simulink model "chap04_CA2"  (R2021a)
settings: Solver=FixedStepDiscrete  StartTime=0.0  StopTime=30  FixedStep=0.001  RelTol=1e-3
undefined symbols (not defined in the file): DiscIntNeverNeededParam
libraries: simulink x4
(part 1 of 3)
settings Model: Creator=陈天兴  LastModifiedBy=陈天兴

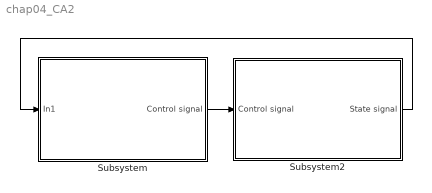
== system chap04_CA2 ==
  Subsystem : Subsystem
  Subsystem2 : Subsystem
  wires:
  Subsystem/1(Control signal) -> Subsystem2/1(Control signal)
  Subsystem2/1(State signal) -> Subsystem/1(In1)

== system chap04_CA2/Subsystem ==
  In1 : Inport
  Bus Creator : BusCreator  Inputs=6
  Bus Creator2 : BusCreator  Inputs=2
  Subsystem : Subsystem
  Subsystem1 : Subsystem
  Subsystem2 : Subsystem
  Subsystem3 : Subsystem
  Subsystem4 : Subsystem
  Subsystem5 : Subsystem
  Control signal : Outport
  wires:
  Bus Creator2/1 -> Subsystem/1(In19), Subsystem2/1(In19), Subsystem5/1(In19), Subsystem4/1(In19), Subsystem1/1(In19), Subsystem3/1(In19)
  Subsystem5/1(u3) -> Bus Creator/3
  Subsystem3/1(u4) -> Bus Creator/4
  Subsystem1/1(u5) -> Bus Creator/5
  Subsystem/1(u1) -> Bus Creator/1
  Subsystem2/1(u2) -> Bus Creator/2
  Subsystem4/1(u6) -> Bus Creator/6
  Bus Creator/1 -> [control], Control signal/1
  In1/1 -> Bus Creator2/1  "state(t)"
  [control] -> Bus Creator2/2  "control"

== system chap04_CA2/Subsystem2 ==
  Control signal : Inport
  Bus Creator : BusCreator  Inputs=7
  Bus Creator1 : BusCreator  Inputs=6
  Bus Selector : BusSelector  OutputSignals=node1.ux,node1.uy,node1.uz
  Bus Selector1 : BusSelector  OutputSignals=node2.ux,node2.uy,node2.uz
  Bus Selector2 : BusSelector  OutputSignals=node3.ux,node3.uy,node3.uz
  Bus Selector3 : BusSelector  OutputSignals=node4.ux,node4.uy,node4.uz
  Bus Selector4 : BusSelector  OutputSignals=node5.ux,node5.uy,node5.uz
  Bus Selector5 : BusSelector  OutputSignals=node6.ux,node6.uy,node6.uz
  Constant2 : Constant
  Scope : Scope  NumInputPorts=3
  Subsystem : Subsystem
  Subsystem1 : Subsystem
  Subsystem2 : Subsystem
  Subsystem3 : Subsystem
  Subsystem4 : Subsystem
  Subsystem5 : Subsystem
  Subsystem6 : Subsystem
  Subsystem7 : Subsystem
  State signal : Outport
  wires:
  Bus Creator/1 -> State signal/1
  Control signal/1 -> Bus Selector/1, Bus Selector1/1, Bus Selector5/1, Bus Selector4/1, Bus Selector3/1, Bus Selector2/1
  Bus Selector/1 -> Subsystem/4(ut1x)  "<ux>"
  Bus Selector/2 -> Subsystem/5(ut1y)  "<uy>"
  Bus Selector/3 -> Subsystem/6(ut1z)  "<uz>"
  Bus Selector1/1 -> Subsystem1/4(ut2x)  "<ux>"
  Bus Selector1/2 -> Subsystem1/5(ut2y)  "<uy>"
  Bus Selector1/3 -> Subsystem1/6(ut2z)  "<uz>"
  Bus Selector2/1 -> Subsystem2/4(ut3x)  "<ux>"
  Bus Selector2/2 -> Subsystem2/5(ut3y)  "<uy>"
  Bus Selector2/3 -> Subsystem2/6(ut3z)  "<uz>"
  Bus Selector3/1 -> Subsystem3/4(ut4x)  "<ux>"
  Bus Selector3/2 -> Subsystem3/5(ut4y)  "<uy>"
  Bus Selector3/3 -> Subsystem3/6(ut4z)  "<uz>"
  Bus Selector4/1 -> Subsystem4/4(ut5x)  "<ux>"
  Bus Selector4/2 -> Subsystem4/5(ut5y)  "<uy>"
  Bus Selector4/3 -> Subsystem4/6(ut5z)  "<uz>"
  Bus Selector5/1 -> Subsystem5/4(ut6x)  "<ux>"
  Bus Selector5/2 -> Subsystem5/5(ut6y)  "<uy>"
  Bus Selector5/3 -> Subsystem5/6(ut6z)  "<uz>"
  Subsystem5/1(node6) -> Bus Creator/7
  Subsystem4/1(node5) -> Bus Creator/6
  Subsystem3/1(node4) -> Bus Creator/5
  Subsystem2/1(node3) -> Bus Creator/4
  Subsystem1/1(node2) -> Bus Creator/3
  Subsystem/1(node1) -> Bus Creator/2
  Subsystem6/5(vy) -> Bus Creator1/5  "vy"
  Subsystem6/2(xy) -> Bus Creator1/2  "xy"
  Subsystem6/3(xz) -> Bus Creator1/3  "xz"
  Subsystem6/4(vx) -> Bus Creator1/4  "vx"
  Subsystem6/6(vz) -> Bus Creator1/6  "vz"
  Bus Creator1/1 -> Bus Creator/1  "node0"
  Subsystem6/1(xx) -> Bus Creator1/1  "xx"
  Subsystem7/2(dy) -> Subsystem/2(dy), Subsystem5/2(dy), Subsystem4/2(dy), Subsystem3/2(dy), Subsystem2/2(dy), Subsystem1/2(dy), Scope/2  "dy"
  Subsystem7/3(dz) -> Subsystem5/3(dz), Subsystem4/3(dz), Subsystem3/3(dz), Subsystem2/3(dz), Subsystem1/3(dz), Subsystem/3(dz), Scope/3  "dz"
  Subsystem7/1(dx) -> Subsystem3/1(dx), Subsystem5/1(dx), Subsystem4/1(dx), Subsystem2/1(dx), Subsystem1/1(dx), Subsystem/1(dx), Scope/1  "dx"
  Constant2/1 -> Subsystem7/1(switch)

== system chap04_CA2/Subsystem/Subsystem ==
  In19 : Inport
  Bus Creator : BusCreator  Inputs=3
  Bus Selector : BusSelector  OutputSignals=state(t).node1.xx,state(t).node2.xx,state(t).node3.xx,state(t).node6.xx,state(t).node1.vx,state(t).node2.vx,state(t).node3.vx,state(t).node6.vx
  Bus Selector1 : BusSelector  OutputSignals=state(t).node1.xy,state(t).node2.xy,state(t).node3.xy,state(t).node6.xy,state(t).node1.vy,state(t).node2.vy,state(t).node3.vy,state(t).node6.vy
  Bus Selector2 : BusSelector  OutputSignals=state(t).node1.xz,state(t).node2.xz,state(t).node3.xz,state(t).node6.xz,state(t).node1.vz,state(t).node2.vz,state(t).node3.vz,state(t).node6.vz
  Bus Selector3 : BusSelector  OutputSignals=state(t).node1.vx
  Bus Selector4 : BusSelector  OutputSignals=state(t).node1.vy
  Bus Selector5 : BusSelector  OutputSignals=state(t).node1.vz
  Constant : Constant  Value=1.5
  Subsystem1 : Subsystem
  Subsystem10 : Subsystem
  Subsystem2 : Subsystem
  Subsystem4 : Subsystem
  Subsystem6 : Subsystem
  Subsystem7 : Subsystem
  Subsystem8 : Subsystem
  u1 : Outport
  wires:
  Subsystem2/1(utx) -> Subsystem8/2(utz)
  Subsystem6/1(utx) -> Subsystem4/2(utx)
  Subsystem1/1(utx) -> Subsystem7/2(uty)
  Bus Creator/1 -> u1/1  "node1"
  [state] -> Bus Selector3/1
  Bus Selector3/1 -> Subsystem4/1(vx1)  "<vx>"
  Bus Selector4/1 -> Subsystem7/1(vy1)  "<vy>"
  [state] -> Bus Selector4/1
  [state] -> Bus Selector5/1
  Bus Selector5/1 -> Subsystem8/1(vz1)  "<vz>"
  [gain] -> Subsystem8/3(gain)
  [gain] -> Subsystem7/3(gain)
  [gain] -> Subsystem4/3(gain)
  Subsystem10/1(ux) -> Bus Creator/1  "ux"
  Subsystem10/2(uy) -> Bus Creator/2  "uy"
  Subsystem10/3(uz) -> Bus Creator/3  "uz"
  In19/1 -> Bus Selector1/1, Bus Selector/1, Bus Selector2/1, [state]
  Bus Selector1/2 -> Subsystem1/2(xy2)  "<xy>"
  Bus Selector/2 -> Subsystem6/2(xx2)  "<xx>"
  Bus Selector/7 -> Subsystem6/7(vx3)  "<vx>"
  Bus Selector2/3 -> Subsystem2/3(xz3)  "<xz>"
  Bus Selector2/6 -> Subsystem2/6(vz2)  "<vz>"
  Bus Selector2/7 -> Subsystem2/7(vz3)  "<vz>"
  Bus Selector/1 -> Subsystem6/1(xx1)  "<xx>"
  Bus Selector1/4 -> Subsystem1/4(xy6)  "<xy>"
  Bus Selector2/5 -> Subsystem2/5(vz1)  "<vz>"
  Bus Selector2/4 -> Subsystem2/4(xz6)  "<xz>"
  Bus Selector/6 -> Subsystem6/6(vx2)  "<vx>"
  Bus Selector1/1 -> Subsystem1/1(xy1)  "<xy>"
  Bus Selector2/8 -> Subsystem2/8(vz6)  "<vz>"
  Bus Selector2/1 -> Subsystem2/1(xz1)  "<xz>"
  Bus Selector2/2 -> Subsystem2/2(xx2)  "<xz>"
  Bus Selector1/8 -> Subsystem1/8(vy6)  "<vy>"
  Bus Selector1/7 -> Subsystem1/7(vy3)  "<vy>"
  Bus Selector1/3 -> Subsystem1/3(xy3)  "<xy>"
  Bus Selector1/5 -> Subsystem1/5(vy1)  "<vy>"
  Bus Selector1/6 -> Subsystem1/6(vy2)  "<vy>"
  Bus Selector/5 -> Subsystem6/5(vx1)  "<vx>"
  Bus Selector/4 -> Subsystem6/4(xx6)  "<xx>"
  Bus Selector/3 -> Subsystem6/3(xx3)  "<xx>"
  Bus Selector/8 -> Subsystem6/8(vx6)  "<vx>"
  Subsystem7/1(ux) -> Subsystem10/2(uty)
  Subsystem4/1(ux) -> Subsystem10/1(utx)
  Subsystem8/1(ux) -> Subsystem10/3(utz)
  Constant/1 -> [gain]

== system chap04_CA2/Subsystem/Subsystem1 ==
  In19 : Inport
  Bus Creator : BusCreator  Inputs=3
  Bus Selector : BusSelector  OutputSignals=state(t).node5.xx,state(t).node0.xx,state(t).node3.xx,state(t).node4.xx,state(t).node5.vx,state(t).node0.vx,state(t).node3.vx,state(t).node4.vx
  Bus Selector1 : BusSelector  OutputSignals=state(t).node5.xy,state(t).node0.xy,state(t).node3.xy,state(t).node4.xy,state(t).node5.vy,state(t).node0.vy,state(t).node3.vy,state(t).node4.vy
  Bus Selector2 : BusSelector  OutputSignals=state(t).node5.xz,state(t).node0.xz,state(t).node3.xz,state(t).node4.xz,state(t).node5.vz,state(t).node0.vz,state(t).node3.vz,state(t).node4.vz
  Bus Selector3 : BusSelector  OutputSignals=state(t).node5.vx,state(t).node0.vx
  Bus Selector4 : BusSelector  OutputSignals=state(t).node5.vy,state(t).node0.vx
  Bus Selector5 : BusSelector  OutputSignals=state(t).node5.vz,state(t).node0.vz
  Constant : Constant  Value=1.5
  Subsystem1 : Subsystem
  Subsystem10 : Subsystem
  Subsystem2 : Subsystem
  Subsystem4 : Subsystem
  Subsystem6 : Subsystem
  Subsystem7 : Subsystem
  Subsystem8 : Subsystem
  u5 : Outport
  wires:
  Bus Creator/1 -> u5/1  "node5"
  Subsystem10/3(uz) -> Bus Creator/3  "uz"
  Subsystem10/2(uy) -> Bus Creator/2  "uy"
  Subsystem10/1(ux) -> Bus Creator/1  "ux"
  [gain] -> Subsystem8/4(gain)
  Subsystem2/1(utz) -> Subsystem8/3(utz)
  Subsystem1/1(uty) -> Subsystem7/3(uty)
  [state] -> Bus Selector3/1
  Bus Selector3/2 -> Subsystem4/2(vx0)  "<vx>"
  Bus Selector3/1 -> Subsystem4/1(vx5)  "<vx>"
  Bus Selector5/1 -> Subsystem8/1(vz5)  "<vz>"
  [state] -> Bus Selector4/1
  Subsystem6/1(utx) -> Subsystem4/3(utx)
  [state] -> Bus Selector5/1
  Bus Selector4/1 -> Subsystem7/1(vy5)  "<vy>"
  Bus Selector4/2 -> Subsystem7/2(vy0)  "<vx>"
  Bus Selector5/2 -> Subsystem8/2(vz0)  "<vz>"
  [gain] -> Subsystem4/4(gain)
  [gain] -> Subsystem7/4(gain)
  In19/1 -> Bus Selector/1, Bus Selector2/1, [state], Bus Selector1/1
  Bus Selector1/8 -> Subsystem1/8(vy4)  "<vy>"
  Bus Selector1/7 -> Subsystem1/7(vy3)  "<vy>"
  Bus Selector1/6 -> Subsystem1/6(vy0)  "<vy>"
  Bus Selector1/5 -> Subsystem1/5(vy5)  "<vy>"
  Bus Selector1/4 -> Subsystem1/4(xy4)  "<xy>"
  Bus Selector1/3 -> Subsystem1/3(xy3)  "<xy>"
  Bus Selector1/2 -> Subsystem1/2(xy0)  "<xy>"
  Bus Selector1/1 -> Subsystem1/1(xy5)  "<xy>"
  Bus Selector/8 -> Subsystem6/8(vx4)  "<vx>"
  Bus Selector/7 -> Subsystem6/7(vx3)  "<vx>"
  Bus Selector/6 -> Subsystem6/6(vx0)  "<vx>"
  Bus Selector/5 -> Subsystem6/5(vx5)  "<vx>"
  Bus Selector/4 -> Subsystem6/4(xx4)  "<xx>"
  Bus Selector/3 -> Subsystem6/3(xx3)  "<xx>"
  Bus Selector/2 -> Subsystem6/2(xx0)  "<xx>"
  Bus Selector/1 -> Subsystem6/1(xx5)  "<xx>"
  Bus Selector2/1 -> Subsystem2/1(xz5)  "<xz>"
  Bus Selector2/2 -> Subsystem2/2(xz0)  "<xz>"
  Bus Selector2/3 -> Subsystem2/3(xz3)  "<xz>"
  Bus Selector2/4 -> Subsystem2/4(xz4)  "<xz>"
  Bus Selector2/5 -> Subsystem2/5(vz5)  "<vz>"
  Bus Selector2/6 -> Subsystem2/6(vz0)  "<vz>"
  Bus Selector2/7 -> Subsystem2/7(vz3)  "<vz>"
  Bus Selector2/8 -> Subsystem2/8(vz4)  "<vz>"
  Subsystem7/1(ux) -> Subsystem10/2(uty)
  Subsystem8/1(ux) -> Subsystem10/3(utz)
  Subsystem4/1(ux) -> Subsystem10/1(utx)
  Constant/1 -> [gain]

== system chap04_CA2/Subsystem/Subsystem2 ==
  In19 : Inport
  Bus Creator : BusCreator  Inputs=3
  Bus Selector10 : BusSelector  OutputSignals=state(t).node2.xy,state(t).node1.xy,state(t).node4.xy,state(t).node6.xy,state(t).node2.vy,state(t).node1.vy,state(t).node4.vy,state(t).node6.vy
  Bus Selector11 : BusSelector  OutputSignals=state(t).node2.xz,state(t).node1.xz,state(t).node4.xz,state(t).node6.xz,state(t).node2.vz,state(t).node1.vz,state(t).node4.vz,state(t).node6.vz
  Bus Selector3 : BusSelector  OutputSignals=state(t).node2.vx
  Bus Selector4 : BusSelector  OutputSignals=state(t).node2.vy
  Bus Selector5 : BusSelector  OutputSignals=state(t).node2.vz
  Bus Selector9 : BusSelector  OutputSignals=state(t).node2.xx,state(t).node1.xx,state(t).node4.xx,state(t).node6.xx,state(t).node2.vx,state(t).node1.vx,state(t).node4.vx,state(t).node6.vx
  Constant : Constant  Value=1.5
  Subsystem1 : Subsystem
  Subsystem10 : Subsystem
  Subsystem2 : Subsystem
  Subsystem4 : Subsystem
  Subsystem6 : Subsystem
  Subsystem7 : Subsystem
  Subsystem8 : Subsystem
  u2 : Outport
  wires:
  Bus Creator/1 -> u2/1  "node2"
  Subsystem10/1(ux) -> Bus Creator/1  "ux"
  Subsystem10/2(uy) -> Bus Creator/2  "uy"
  Subsystem10/3(uz) -> Bus Creator/3  "uz"
  Subsystem1/1(p2y) -> Subsystem7/2(uty)
  [state] -> Bus Selector4/1
  Subsystem2/1(p2z) -> Subsystem8/2(utz)
  Bus Selector4/1 -> Subsystem7/1(vy1)  "<vy>"
  Bus Selector5/1 -> Subsystem8/1(vz1)  "<vz>"
  [gain] -> Subsystem8/3(gain)
  [gain] -> Subsystem4/3(gain)
  [gain] -> Subsystem7/3(gain)
  [state] -> Bus Selector3/1
  Subsystem6/1(p2x) -> Subsystem4/2(utx)
  Bus Selector3/1 -> Subsystem4/1(vx1)  "<vx>"
  [state] -> Bus Selector5/1
  Bus Selector11/8 -> Subsystem2/8(vz6)  "<vz>"
  Bus Selector11/7 -> Subsystem2/7(vz4)  "<vz>"
  Bus Selector11/6 -> Subsystem2/6(vz1)  "<vz>"
  Bus Selector11/5 -> Subsystem2/5(vz2)  "<vz>"
  Bus Selector11/4 -> Subsystem2/4(xz6)  "<xz>"
  Bus Selector11/3 -> Subsystem2/3(xz4)  "<xz>"
  Bus Selector11/2 -> Subsystem2/2(xz1)  "<xz>"
  Bus Selector11/1 -> Subsystem2/1(xz2)  "<xz>"
  Bus Selector10/8 -> Subsystem1/8(vy6)  "<vy>"
  Bus Selector10/7 -> Subsystem1/7(vy4)  "<vy>"
  Bus Selector10/6 -> Subsystem1/6(vy1)  "<vy>"
  Bus Selector10/5 -> Subsystem1/5(vy2)  "<vy>"
  Bus Selector10/4 -> Subsystem1/4(xy6)  "<xy>"
  Bus Selector10/3 -> Subsystem1/3(xy4)  "<xy>"
  Bus Selector10/2 -> Subsystem1/2(xy1)  "<xy>"
  Bus Selector10/1 -> Subsystem1/1(xy2)  "<xy>"
  Bus Selector9/1 -> Subsystem6/1(xx2)  "<xx>"
  Bus Selector9/2 -> Subsystem6/2(xx1)  "<xx>"
  Bus Selector9/3 -> Subsystem6/3(xx4)  "<xx>"
  Bus Selector9/4 -> Subsystem6/4(xx6)  "<xx>"
  Bus Selector9/5 -> Subsystem6/5(vx2)  "<vx>"
  Bus Selector9/6 -> Subsystem6/6(vx1)  "<vx>"
  Bus Selector9/7 -> Subsystem6/7(vx4)  "<vx>"
  Bus Selector9/8 -> Subsystem6/8(vx6)  "<vx>"
  In19/1 -> [state], Bus Selector11/1, Bus Selector9/1, Bus Selector10/1
  Subsystem7/1(ux) -> Subsystem10/2(uty)
  Subsystem8/1(ux) -> Subsystem10/3(utz)
  Subsystem4/1(ux) -> Subsystem10/1(utx)
  Constant/1 -> [gain]

== system chap04_CA2/Subsystem/Subsystem3 ==
  In19 : Inport
  Bus Creator : BusCreator  Inputs=3
  Bus Selector : BusSelector  OutputSignals=state(t).node4.xx,state(t).node2.xx,state(t).node3.xx,state(t).node5.xx,state(t).node4.vx,state(t).node2.vx,state(t).node3.vx,state(t).node5.vx
  Bus Selector1 : BusSelector  OutputSignals=state(t).node4.xy,state(t).node2.xy,state(t).node3.xy,state(t).node5.xy,state(t).node4.vy,state(t).node2.vy,state(t).node3.vy,state(t).node5.vy
  Bus Selector2 : BusSelector  OutputSignals=state(t).node4.xz,state(t).node2.xz,state(t).node3.xz,state(t).node5.xz,state(t).node4.vz,state(t).node2.vz,state(t).node3.vz,state(t).node5.vz
  Bus Selector3 : BusSelector  OutputSignals=state(t).node4.vx
  Bus Selector4 : BusSelector  OutputSignals=state(t).node4.vy
  Bus Selector5 : BusSelector  OutputSignals=state(t).node4.vz
  Constant : Constant  Value=1.5
  Subsystem1 : Subsystem
  Subsystem10 : Subsystem
  Subsystem2 : Subsystem
  Subsystem4 : Subsystem
  Subsystem6 : Subsystem
  Subsystem7 : Subsystem
  Subsystem8 : Subsystem
  u4 : Outport
  wires:
  Bus Creator/1 -> u4/1  "node4"
  [state] -> Bus Selector5/1
  Subsystem2/1(utx) -> Subsystem8/2(utz)
  Bus Selector5/1 -> Subsystem8/1(vz4)  "<vz>"
  [state] -> Bus Selector4/1
  [gain] -> Subsystem8/3(gain)
  Subsystem6/1(utx) -> Subsystem4/2(utx)
  Bus Selector4/1 -> Subsystem7/1(vy4)  "<vy>"
  Subsystem1/1(utx) -> Subsystem7/2(uty)
  Bus Selector3/1 -> Subsystem4/1(vx4)  "<vx>"
  [gain] -> Subsystem7/3(gain)
  [gain] -> Subsystem4/3(gain)
  [state] -> Bus Selector3/1
  Subsystem10/1(ux) -> Bus Creator/1  "ux"
  Subsystem10/2(uy) -> Bus Creator/2  "uy"
  Subsystem10/3(uz) -> Bus Creator/3  "uz"
  Bus Selector1/6 -> Subsystem1/6(vy2)  "<vy>"
  Bus Selector/6 -> Subsystem6/6(vx2)  "<vx>"
  In19/1 -> Bus Selector/1, Bus Selector1/1, Bus Selector2/1, [state]
  Bus Selector/7 -> Subsystem6/7(vx3)  "<vx>"
  Bus Selector1/2 -> Subsystem1/2(xy2)  "<xy>"
  Bus Selector2/3 -> Subsystem2/3(xz3)  "<xz>"
  Bus Selector1/3 -> Subsystem1/3(xy3)  "<xy>"
  Bus Selector2/1 -> Subsystem2/1(xz4)  "<xz>"
  Bus Selector1/1 -> Subsystem1/1(xy4)  "<xy>"
  Bus Selector/3 -> Subsystem6/3(xx3)  "<xx>"
  Bus Selector/1 -> Subsystem6/1(xx4)  "<xx>"
  Bus Selector/8 -> Subsystem6/8(vx5)  "<vx>"
  Bus Selector1/4 -> Subsystem1/4(xy5)  "<xy>"
  Bus Selector/4 -> Subsystem6/4(xx5)  "<xx>"
  Bus Selector/5 -> Subsystem6/5(vx4)  "<vx>"
  Bus Selector1/7 -> Subsystem1/7(vy3)  "<vy>"
  Bus Selector2/7 -> Subsystem2/7(vz3)  "<vz>"
  Bus Selector2/4 -> Subsystem2/4(xz5)  "<xz>"
  Bus Selector2/8 -> Subsystem2/8(vz5)  "<vz>"
  Bus Selector1/8 -> Subsystem1/8(vy5)  "<vy>"
  Bus Selector/2 -> Subsystem6/2(xx2)  "<xx>"
  Bus Selector2/2 -> Subsystem2/2(xx2)  "<xz>"
  Bus Selector1/5 -> Subsystem1/5(vy4)  "<vy>"
  Bus Selector2/5 -> Subsystem2/5(vz4)  "<vz>"
  Bus Selector2/6 -> Subsystem2/6(vz2)  "<vz>"
  Subsystem4/1(ux) -> Subsystem10/1(utx)
  Subsystem8/1(ux) -> Subsystem10/3(utz)
  Subsystem7/1(ux) -> Subsystem10/2(uty)
  Constant/1 -> [gain]

== system chap04_CA2/Subsystem/Subsystem4 ==
  In19 : Inport
  Bus Creator : BusCreator  Inputs=3
  Bus Selector : BusSelector  OutputSignals=state(t).node6.xx,state(t).node0.xx,state(t).node1.xx,state(t).node2.xx,state(t).node6.vx,state(t).node0.vx,state(t).node1.vx,state(t).node2.vx
  Bus Selector1 : BusSelector  OutputSignals=state(t).node6.xy,state(t).node0.xy,state(t).node1.xy,state(t).node2.xy,state(t).node6.vy,state(t).node0.vy,state(t).node1.vy,state(t).node2.vy
  Bus Selector2 : BusSelector  OutputSignals=state(t).node6.xz,state(t).node0.xz,state(t).node1.xz,state(t).node2.xz,state(t).node6.vz,state(t).node0.vz,state(t).node1.vz,state(t).node2.vz
  Bus Selector3 : BusSelector  OutputSignals=state(t).node6.vx,state(t).node0.vx
  Bus Selector4 : BusSelector  OutputSignals=state(t).node6.vy,state(t).node0.vx
  Bus Selector5 : BusSelector  OutputSignals=state(t).node6.vz,state(t).node0.vz
  Constant : Constant  Value=1.5
  Subsystem1 : Subsystem
  Subsystem10 : Subsystem
  Subsystem2 : Subsystem
  Subsystem4 : Subsystem
  Subsystem6 : Subsystem
  Subsystem7 : Subsystem
  Subsystem8 : Subsystem
  u6 : Outport
  wires:
  Bus Creator/1 -> u6/1  "node6"
  Subsystem10/3(uz) -> Bus Creator/3  "uz"
  Subsystem10/2(uy) -> Bus Creator/2  "uy"
  Subsystem10/1(ux) -> Bus Creator/1  "ux"
  Bus Selector5/2 -> Subsystem8/2(vz0)  "<vz>"
  [gain] -> Subsystem7/4(gain)
  Subsystem1/1(utx) -> Subsystem7/3(uty)
  Subsystem2/1(utx) -> Subsystem8/3(utz)
  [state] -> Bus Selector3/1
  Bus Selector5/1 -> Subsystem8/1(vz6)  "<vz>"
  Bus Selector4/2 -> Subsystem7/2(vy0)  "<vx>"
  [gain] -> Subsystem4/4(gain)
  [state] -> Bus Selector5/1
  Subsystem6/1(utx) -> Subsystem4/3(utx)
  Bus Selector3/1 -> Subsystem4/1(vx6)  "<vx>"
  Bus Selector3/2 -> Subsystem4/2(vx0)  "<vx>"
  [gain] -> Subsystem8/4(gain)
  [state] -> Bus Selector4/1
  Bus Selector4/1 -> Subsystem7/1(vy6)  "<vy>"
  In19/1 -> Bus Selector/1, [state], Bus Selector2/1, Bus Selector1/1
  Bus Selector1/1 -> Subsystem1/1(xx6)  "<xy>"
  Bus Selector1/2 -> Subsystem1/2(xx0)  "<xy>"
  Bus Selector1/3 -> Subsystem1/3(xx1)  "<xy>"
  Bus Selector1/4 -> Subsystem1/4(xx2)  "<xy>"
  Bus Selector1/5 -> Subsystem1/5(vx6)  "<vy>"
  Bus Selector1/6 -> Subsystem1/6(vx0)  "<vy>"
  Bus Selector1/7 -> Subsystem1/7(vx1)  "<vy>"
  Bus Selector1/8 -> Subsystem1/8(vx2)  "<vy>"
  Bus Selector2/1 -> Subsystem2/1(xx6)  "<xz>"
  Bus Selector2/3 -> Subsystem2/3(xx1)  "<xz>"
  Bus Selector2/2 -> Subsystem2/2(xx0)  "<xz>"
  Bus Selector2/4 -> Subsystem2/4(xx2)  "<xz>"
  Bus Selector2/5 -> Subsystem2/5(vx6)  "<vz>"
  Bus Selector2/6 -> Subsystem2/6(vx0)  "<vz>"
  Bus Selector2/7 -> Subsystem2/7(vx1)  "<vz>"
  Bus Selector2/8 -> Subsystem2/8(vx2)  "<vz>"
  Bus Selector/8 -> Subsystem6/8(vx2)  "<vx>"
  Bus Selector/7 -> Subsystem6/7(vx1)  "<vx>"
  Bus Selector/6 -> Subsystem6/6(vx0)  "<vx>"
  Bus Selector/5 -> Subsystem6/5(vx6)  "<vx>"
  Bus Selector/4 -> Subsystem6/4(xx2)  "<xx>"
  Bus Selector/3 -> Subsystem6/3(xx1)  "<xx>"
  Bus Selector/2 -> Subsystem6/2(xx0)  "<xx>"
  Bus Selector/1 -> Subsystem6/1(xx6)  "<xx>"
  Subsystem7/1(ux) -> Subsystem10/2(uty)
  Subsystem8/1(ux) -> Subsystem10/3(utz)
  Subsystem4/1(ux) -> Subsystem10/1(utx)
  Constant/1 -> [gain]

== system chap04_CA2/Subsystem/Subsystem5 ==
  In19 : Inport
  Bus Creator : BusCreator  Inputs=3
  Bus Selector10 : BusSelector  OutputSignals=state(t).node3.xy,state(t).node1.xy,state(t).node4.xy,state(t).node5.xy,state(t).node3.vy,state(t).node1.vy,state(t).node4.vy,state(t).node5.vy
  Bus Selector11 : BusSelector  OutputSignals=state(t).node3.xz,state(t).node1.xz,state(t).node4.xz,state(t).node5.xz,state(t).node3.vz,state(t).node1.vz,state(t).node4.vz,state(t).node5.vz
  Bus Selector3 : BusSelector  OutputSignals=state(t).node3.vx
  Bus Selector4 : BusSelector  OutputSignals=state(t).node3.vy
  Bus Selector5 : BusSelector  OutputSignals=state(t).node3.vz
  Bus Selector9 : BusSelector  OutputSignals=state(t).node3.xx,state(t).node1.xx,state(t).node4.xx,state(t).node5.xx,state(t).node3.vx,state(t).node1.vx,state(t).node4.vx,state(t).node5.vx
  Constant : Constant  Value=1.5
  Subsystem1 : Subsystem
  Subsystem10 : Subsystem
  Subsystem2 : Subsystem
  Subsystem4 : Subsystem
  Subsystem6 : Subsystem
  Subsystem7 : Subsystem
  Subsystem8 : Subsystem
  u3 : Outport
  wires:
  Bus Creator/1 -> u3/1  "node3"
  Subsystem10/1(ux) -> Bus Creator/1  "ux"
  Subsystem10/2(uy) -> Bus Creator/2  "uy"
  Subsystem10/3(uz) -> Bus Creator/3  "uz"
  In19/1 -> Bus Selector9/1, Bus Selector10/1, [state], Bus Selector11/1
  Subsystem6/1(p3x) -> Subsystem4/2(utx)
  [gain] -> Subsystem7/3(gain)
  Bus Selector4/1 -> Subsystem7/1(vy3)  "<vy>"
  [state] -> Bus Selector5/1
  [state] -> Bus Selector3/1
  Bus Selector3/1 -> Subsystem4/1(vx3)  "<vx>"
  Bus Selector5/1 -> Subsystem8/1(vz3)  "<vz>"
  [gain] -> Subsystem4/3(gain)
  [gain] -> Subsystem8/3(gain)
  Subsystem2/1(p3z) -> Subsystem8/2(utz)
  Subsystem1/1(p3y) -> Subsystem7/2(uty)
  [state] -> Bus Selector4/1
  Bus Selector10/1 -> Subsystem1/1(xy3)  "<xy>"
  Bus Selector10/2 -> Subsystem1/2(xy1)  "<xy>"
  Bus Selector10/3 -> Subsystem1/3(xy4)  "<xy>"
  Bus Selector10/4 -> Subsystem1/4(xy5)  "<xy>"
  Bus Selector10/5 -> Subsystem1/5(vy3)  "<vy>"
  Bus Selector10/6 -> Subsystem1/6(vy1)  "<vy>"
  Bus Selector10/7 -> Subsystem1/7(vy4)  "<vy>"
  Bus Selector10/8 -> Subsystem1/8(vy5)  "<vy>"
  Bus Selector11/1 -> Subsystem2/1(xz3)  "<xz>"
  Bus Selector11/2 -> Subsystem2/2(xz1)  "<xz>"
  Bus Selector11/3 -> Subsystem2/3(xz4)  "<xz>"
  Bus Selector11/4 -> Subsystem2/4(xz5)  "<xz>"
  Bus Selector11/5 -> Subsystem2/5(vz3)  "<vz>"
  Bus Selector11/6 -> Subsystem2/6(vz1)  "<vz>"
  Bus Selector11/7 -> Subsystem2/7(vz4)  "<vz>"
  Bus Selector11/8 -> Subsystem2/8(vz5)  "<vz>"
  Bus Selector9/1 -> Subsystem6/1(xx3)  "<xx>"
  Bus Selector9/2 -> Subsystem6/2(xx1)  "<xx>"
  Bus Selector9/3 -> Subsystem6/3(xx4)  "<xx>"
  Bus Selector9/4 -> Subsystem6/4(xx5)  "<xx>"
  Bus Selector9/5 -> Subsystem6/5(vx3)  "<vx>"
  Bus Selector9/6 -> Subsystem6/6(vx1)  "<vx>"
  Bus Selector9/7 -> Subsystem6/7(vx4)  "<vx>"
  Bus Selector9/8 -> Subsystem6/8(vx5)  "<vx>"
  Subsystem7/1(ux) -> Subsystem10/2(uty)
  Subsystem8/1(ux) -> Subsystem10/3(utz)
  Subsystem4/1(ux) -> Subsystem10/1(utx)
  Constant/1 -> [gain]

== system chap04_CA2/Subsystem2/Subsystem ==
  dx : Inport
  dy : Inport  Port=2
  dz : Inport  Port=3
  ut1x : Inport  Port=4
  ut1y : Inport  Port=5
  ut1z : Inport  Port=6
  Add : Sum
  Add1 : Sum
  Add2 : Sum
  Add3 : Sum  Inputs=-+
  Add4 : Sum  Inputs=-+
  Add5 : Sum  Inputs=-+
  Bus Creator1 : BusCreator  Inputs=6
  Constant : Constant  Value=-1
  Constant1 : Constant
  Constant2 : Constant  Value=0
  Discrete-Time Integrator{,15..17} (4 alike) : DiscreteIntegrator  SampleTime=-1  ICPrevOutput=DiscIntNeverNeededParam  ICPrevScaledInput=DiscIntNeverNeededParam
  Discrete-Time Integrator14 : DiscreteIntegrator  InitialCondition=-1  SampleTime=-1  ICPrevOutput=DiscIntNeverNeededParam  ICPrevScaledInput=DiscIntNeverNeededParam
  Discrete-Time Integrator5 : DiscreteIntegrator  InitialCondition=1  SampleTime=-1  ICPrevOutput=DiscIntNeverNeededParam  ICPrevScaledInput=DiscIntNeverNeededParam
  node1 : Outport
  wires:
  ut1y/1 -> Add1/2
  ut1z/1 -> Add2/2
  Discrete-Time Integrator17/1 -> Discrete-Time Integrator15/1, Bus Creator1/5  "vy"
  Discrete-Time Integrator/1 -> Discrete-Time Integrator5/1, Bus Creator1/6  "vz"
  ut1x/1 -> Add/2
  Discrete-Time Integrator16/1 -> Bus Creator1/4, Discrete-Time Integrator14/1  "vx"
  Bus Creator1/1 -> node1/1  "node1"
  Add5/1 -> Bus Creator1/3  "xz"
  Add4/1 -> Bus Creator1/2  "xy"
  Add3/1 -> Bus Creator1/1  "xx"
  Add/1 -> Discrete-Time Integrator16/1
  Add1/1 -> Discrete-Time Integrator17/1
  Add2/1 -> Discrete-Time Integrator/1
  dy/1 -> Add1/1
  dz/1 -> Add2/1
  dx/1 -> Add/1
  Discrete-Time Integrator14/1 -> Add3/2
  Discrete-Time Integrator5/1 -> Add5/2
  Discrete-Time Integrator15/1 -> Add4/2
  Constant/1 -> Add3/1
  Constant1/1 -> Add4/1
  Constant2/1 -> Add5/1

== system chap04_CA2/Subsystem2/Subsystem1 ==
  dx : Inport
  dy : Inport  Port=2
  dz : Inport  Port=3
  ut2x : Inport  Port=4
  ut2y : Inport  Port=5
  ut2z : Inport  Port=6
  Add : Sum
  Add1 : Sum
  Add2 : Sum
  Add3 : Sum  Inputs=-+
  Add4 : Sum  Inputs=-+
  Add5 : Sum  Inputs=-+
  Bus Creator1 : BusCreator  Inputs=6
  Constant : Constant
  Constant1 : Constant
  Constant2 : Constant  Value=0
  Discrete-Time Integrator : DiscreteIntegrator  SampleTime=-1  ICPrevOutput=DiscIntNeverNeededParam  ICPrevScaledInput=DiscIntNeverNeededParam
  Discrete-Time Integrator14 : DiscreteIntegrator  InitialCondition=1.5  SampleTime=-1  ICPrevOutput=DiscIntNeverNeededParam  ICPrevScaledInput=DiscIntNeverNeededParam
  Discrete-Time Integrator15 : DiscreteIntegrator  InitialCondition=0.5  SampleTime=-1  ICPrevOutput=DiscIntNeverNeededParam  ICPrevScaledInput=DiscIntNeverNeededParam
  Discrete-Time Integrator16 : DiscreteIntegrator  SampleTime=-1  ICPrevOutput=DiscIntNeverNeededParam  ICPrevScaledInput=DiscIntNeverNeededParam
  Discrete-Time Integrator17 : DiscreteIntegrator  SampleTime=-1  ICPrevOutput=DiscIntNeverNeededParam  ICPrevScaledInput=DiscIntNeverNeededParam
  Discrete-Time Integrator5 : DiscreteIntegrator  InitialCondition=1  SampleTime=-1  ICPrevOutput=DiscIntNeverNeededParam  ICPrevScaledInput=DiscIntNeverNeededParam
  node2 : Outport
  wires:
  Bus Creator1/1 -> node2/1  "node2"
  Discrete-Time Integrator16/1 -> Bus Creator1/4, Discrete-Time Integrator14/1  "vx"
  Discrete-Time Integrator/1 -> Discrete-Time Integrator5/1, Bus Creator1/6  "vz"
  Discrete-Time Integrator17/1 -> Bus Creator1/5, Discrete-Time Integrator15/1  "vy"
  dx/1 -> Add/1
  dy/1 -> Add1/1
  dz/1 -> Add2/1
  Add2/1 -> Discrete-Time Integrator/1
  Add1/1 -> Discrete-Time Integrator17/1
  Add/1 -> Discrete-Time Integrator16/1
  ut2x/1 -> Add/2
  ut2y/1 -> Add1/2
  ut2z/1 -> Add2/2
  Constant2/1 -> Add5/1
  Constant1/1 -> Add4/1
  Discrete-Time Integrator14/1 -> Add3/2
  Discrete-Time Integrator15/1 -> Add4/2
  Discrete-Time Integrator5/1 -> Add5/2
  Constant/1 -> Add3/1
  Add3/1 -> Bus Creator1/1  "xx"
  Add4/1 -> Bus Creator1/2  "xy"
  Add5/1 -> Bus Creator1/3  "xz"

== system chap04_CA2/Subsystem2/Subsystem2 ==
  dx : Inport
  dy : Inport  Port=2
  dz : Inport  Port=3
  ut3x : Inport  Port=4
  ut3y : Inport  Port=5
  ut3z : Inport  Port=6
  Add : Sum
  Add1 : Sum
  Add2 : Sum
  Add3 : Sum  Inputs=-+
  Add4 : Sum  Inputs=-+
  Add5 : Sum  Inputs=-+
  Bus Creator1 : BusCreator  Inputs=6
  Constant : Constant  Value=-2
  Constant1 : Constant  Value=0
  Constant2 : Constant  Value=0
  Discrete-Time Integrator : DiscreteIntegrator  SampleTime=-1  ICPrevOutput=DiscIntNeverNeededParam  ICPrevScaledInput=DiscIntNeverNeededParam
  Discrete-Time Integrator14 : DiscreteIntegrator  InitialCondition=-1  SampleTime=-1  ICPrevOutput=DiscIntNeverNeededParam  ICPrevScaledInput=DiscIntNeverNeededParam
  Discrete-Time Integrator15 : DiscreteIntegrator  InitialCondition=-1  SampleTime=-1  ICPrevOutput=DiscIntNeverNeededParam  ICPrevScaledInput=DiscIntNeverNeededParam
  Discrete-Time Integrator16 : DiscreteIntegrator  SampleTime=-1  ICPrevOutput=DiscIntNeverNeededParam  ICPrevScaledInput=DiscIntNeverNeededParam
  Discrete-Time Integrator17 : DiscreteIntegrator  SampleTime=-1  ICPrevOutput=DiscIntNeverNeededParam  ICPrevScaledInput=DiscIntNeverNeededParam
  Discrete-Time Integrator5 : DiscreteIntegrator  InitialCondition=0.5  SampleTime=-1  ICPrevOutput=DiscIntNeverNeededParam  ICPrevScaledInput=DiscIntNeverNeededParam
  node3 : Outport
  wires:
  Discrete-Time Integrator17/1 -> Discrete-Time Integrator15/1, Bus Creator1/5  "vy"
  Discrete-Time Integrator/1 -> Discrete-Time Integrator5/1, Bus Creator1/6  "vz"
  Discrete-Time Integrator16/1 -> Bus Creator1/4, Discrete-Time Integrator14/1  "vx"
  Bus Creator1/1 -> node3/1  "node3"
  ut3x/1 -> Add/2
  ut3y/1 -> Add1/2
  Add/1 -> Discrete-Time Integrator16/1
  dy/1 -> Add1/1
  Add1/1 -> Discrete-Time Integrator17/1
  Add2/1 -> Discrete-Time Integrator/1
  dz/1 -> Add2/1
  dx/1 -> Add/1
  ut3z/1 -> Add2/2
  Constant2/1 -> Add5/1
  Constant1/1 -> Add4/1
  Discrete-Time Integrator14/1 -> Add3/2
  Discrete-Time Integrator15/1 -> Add4/2
  Discrete-Time Integrator5/1 -> Add5/2
  Constant/1 -> Add3/1
  Add3/1 -> Bus Creator1/1  "xx"
  Add4/1 -> Bus Creator1/2  "xy"
  Add5/1 -> Bus Creator1/3  "xz"

== system chap04_CA2/Subsystem2/Subsystem3 ==
  dx : Inport
  dy : Inport  Port=2
  dz : Inport  Port=3
  ut4x : Inport  Port=4
  ut4y : Inport  Port=5
  ut4z : Inport  Port=6
  Add : Sum
  Add1 : Sum
  Add2 : Sum
  Add3 : Sum  Inputs=-+
  Add4 : Sum  Inputs=-+
  Add5 : Sum  Inputs=-+
  Bus Creator1 : BusCreator  Inputs=6
  Constant : Constant  Value=2
  Constant1 : Constant  Value=0
  Constant2 : Constant  Value=0
  Discrete-Time Integrator : DiscreteIntegrator  SampleTime=-1  ICPrevOutput=DiscIntNeverNeededParam  ICPrevScaledInput=DiscIntNeverNeededParam
  Discrete-Time Integrator14 : DiscreteIntegrator  InitialCondition=4  SampleTime=-1  ICPrevOutput=DiscIntNeverNeededParam  ICPrevScaledInput=DiscIntNeverNeededParam
  Discrete-Time Integrator15 : DiscreteIntegrator  InitialCondition=-1  SampleTime=-1  ICPrevOutput=DiscIntNeverNeededParam  ICPrevScaledInput=DiscIntNeverNeededParam
  Discrete-Time Integrator16 : DiscreteIntegrator  SampleTime=-1  ICPrevOutput=DiscIntNeverNeededParam  ICPrevScaledInput=DiscIntNeverNeededParam
  Discrete-Time Integrator17 : DiscreteIntegrator  SampleTime=-1  ICPrevOutput=DiscIntNeverNeededParam  ICPrevScaledInput=DiscIntNeverNeededParam
  Discrete-Time Integrator5 : DiscreteIntegrator  InitialCondition=0.5  SampleTime=-1  ICPrevOutput=DiscIntNeverNeededParam  ICPrevScaledInput=DiscIntNeverNeededParam
  node4 : Outport
  wires:
  Bus Creator1/1 -> node4/1  "node4"
  Discrete-Time Integrator16/1 -> Discrete-Time Integrator14/1, Bus Creator1/4  "vx"
  Discrete-Time Integrator/1 -> Discrete-Time Integrator5/1, Bus Creator1/6  "vz"
  Discrete-Time Integrator17/1 -> Bus Creator1/5, Discrete-Time Integrator15/1  "vy"
  ut4x/1 -> Add/2
  ut4y/1 -> Add1/2
  Add/1 -> Discrete-Time Integrator16/1
  dy/1 -> Add1/1
  Add1/1 -> Discrete-Time Integrator17/1
  Add2/1 -> Discrete-Time Integrator/1
  dz/1 -> Add2/1
  dx/1 -> Add/1
  ut4z/1 -> Add2/2
  Constant2/1 -> Add5/1
  Constant1/1 -> Add4/1
  Discrete-Time Integrator14/1 -> Add3/2
  Discrete-Time Integrator15/1 -> Add4/2
  Discrete-Time Integrator5/1 -> Add5/2
  Constant/1 -> Add3/1
  Add3/1 -> Bus Creator1/1  "xx"
  Add4/1 -> Bus Creator1/2  "xy"
  Add5/1 -> Bus Creator1/3  "xz"

== system chap04_CA2/Subsystem2/Subsystem4 ==
  dx : Inport
  dy : Inport  Port=2
  dz : Inport  Port=3
  ut5x : Inport  Port=4
  ut5y : Inport  Port=5
  ut5z : Inport  Port=6
  Add : Sum
  Add1 : Sum
  Add2 : Sum
  Add3 : Sum  Inputs=-+
  Add4 : Sum  Inputs=-+
  Add5 : Sum  Inputs=-+
  Bus Creator1 : BusCreator  Inputs=6
  Constant : Constant  Value=-1
  Constant1 : Constant  Value=-1
  Constant2 : Constant  Value=0
  Discrete-Time Integrator{,5,16..17} (4 alike) : DiscreteIntegrator  SampleTime=-1  ICPrevOutput=DiscIntNeverNeededParam  ICPrevScaledInput=DiscIntNeverNeededParam
  Discrete-Time Integrator14 : DiscreteIntegrator  InitialCondition=0.7  SampleTime=-1  ICPrevOutput=DiscIntNeverNeededParam  ICPrevScaledInput=DiscIntNeverNeededParam
  Discrete-Time Integrator15 : DiscreteIntegrator  InitialCondition=-1.7  SampleTime=-1  ICPrevOutput=DiscIntNeverNeededParam  ICPrevScaledInput=DiscIntNeverNeededParam
  node5 : Outport
  wires:
  Discrete-Time Integrator17/1 -> Discrete-Time Integrator15/1, Bus Creator1/5  "vy"
  Discrete-Time Integrator/1 -> Discrete-Time Integrator5/1, Bus Creator1/6  "vz"
  Discrete-Time Integrator16/1 -> Bus Creator1/4, Discrete-Time Integrator14/1  "vx"
  Bus Creator1/1 -> node5/1  "node5"
  ut5x/1 -> Add/2
  ut5y/1 -> Add1/2
  Add/1 -> Discrete-Time Integrator16/1
  dy/1 -> Add1/1
  Add1/1 -> Discrete-Time Integrator17/1
  Add2/1 -> Discrete-Time Integrator/1
  dz/1 -> Add2/1
  dx/1 -> Add/1
  ut5z/1 -> Add2/2
  Constant2/1 -> Add5/1
  Constant1/1 -> Add4/1
  Discrete-Time Integrator14/1 -> Add3/2
  Discrete-Time Integrator15/1 -> Add4/2
  Discrete-Time Integrator5/1 -> Add5/2
  Constant/1 -> Add3/1
  Add3/1 -> Bus Creator1/1  "xx"
  Add4/1 -> Bus Creator1/2  "xy"
  Add5/1 -> Bus Creator1/3  "xz"

== system chap04_CA2/Subsystem2/Subsystem5 ==
  dx : Inport
  dy : Inport  Port=2
  dz : Inport  Port=3
  ut6x : Inport  Port=4
  ut6y : Inport  Port=5
  ut6z : Inport  Port=6
  Add : Sum
  Add1 : Sum
  Add2 : Sum
  Add3 : Sum  Inputs=-+
  Add4 : Sum  Inputs=-+
  Add5 : Sum  Inputs=-+
  Bus Creator1 : BusCreator  Inputs=6
  Constant : Constant
  Constant1 : Constant  Value=-1
  Constant2 : Constant  Value=0
  Discrete-Time Integrator{,5,16..17} (4 alike) : DiscreteIntegrator  SampleTime=-1  ICPrevOutput=DiscIntNeverNeededParam  ICPrevScaledInput=DiscIntNeverNeededParam
  Discrete-Time Integrator14 : DiscreteIntegrator  InitialCondition=3  SampleTime=-1  ICPrevOutput=DiscIntNeverNeededParam  ICPrevScaledInput=DiscIntNeverNeededParam
  Discrete-Time Integrator15 : DiscreteIntegrator  InitialCondition=-1.5  SampleTime=-1  ICPrevOutput=DiscIntNeverNeededParam  ICPrevScaledInput=DiscIntNeverNeededParam
  node6 : Outport
  wires:
  Bus Creator1/1 -> node6/1  "node6"
  Discrete-Time Integrator16/1 -> Discrete-Time Integrator14/1, Bus Creator1/4  "vx"
  Discrete-Time Integrator/1 -> Discrete-Time Integrator5/1, Bus Creator1/6  "vz"
  Discrete-Time Integrator17/1 -> Bus Creator1/5, Discrete-Time Integrator15/1  "vy"
  ut6x/1 -> Add/2
  ut6y/1 -> Add1/2
  Add/1 -> Discrete-Time Integrator16/1
  dy/1 -> Add1/1
  Add1/1 -> Discrete-Time Integrator17/1
  Add2/1 -> Discrete-Time Integrator/1
  dz/1 -> Add2/1
  dx/1 -> Add/1
  ut6z/1 -> Add2/2
  Constant2/1 -> Add5/1
  Constant1/1 -> Add4/1
  Discrete-Time Integrator14/1 -> Add3/2
  Discrete-Time Integrator15/1 -> Add4/2
  Discrete-Time Integrator5/1 -> Add5/2
  Constant/1 -> Add3/1
  Add3/1 -> Bus Creator1/1  "xx"
  Add4/1 -> Bus Creator1/2  "xy"
  Add5/1 -> Bus Creator1/3  "xz"

== system chap04_CA2/Subsystem2/Subsystem6 ==
  Clock1 : Clock
  Constant1 : Constant  Value=0.25
  Constant3 : Constant  Value=0.25
  Constant9 : Constant  Value=0.1
  Discrete Derivative : simulink/Discrete/Discrete Derivative  gainval=1.0  ICPrevScaledInput=1000  OutMin=[]  OutMax=[]  OutDataType=fixdt(1, 16)  OutScaling=2^-10  DoSatur=off
  Discrete Derivative1 : simulink/Discrete/Discrete Derivative  gainval=1.0  ICPrevScaledInput=-0.25  OutMin=[]  OutMax=[]  OutDataType=fixdt(1, 16)  OutScaling=2^-10  DoSatur=off
  Discrete Derivative2 : simulink/Discrete/Discrete Derivative  gainval=1.0  ICPrevScaledInput=249.9  OutMin=[]  OutMax=[]  OutDataType=fixdt(1, 16)  OutScaling=2^-10  DoSatur=off
  Product{,1..3} (4 alike) : Product
  Sum : Sum  Inputs=|++
  Trigonometric Function2 : Trigonometry
  Trigonometric Function3 : Trigonometry  Operator=cos
  r : Constant
  xx : Outport
  xy : Outport  Port=2
  xz : Outport  Port=3
  vx : Outport  Port=4
  vy : Outport  Port=5
  vz : Outport  Port=6
  wires:
  Discrete Derivative/1 -> vx/1
  Discrete Derivative1/1 -> vy/1
  Sum/1 -> Discrete Derivative2/1, xz/1
  Discrete Derivative2/1 -> vz/1
  Product/1 -> xx/1, Discrete Derivative/1
  Product1/1 -> xy/1, Discrete Derivative1/1
  Product2/1 -> Trigonometric Function2/1, Trigonometric Function3/1
  Trigonometric Function3/1 -> Product/1
  Constant9/1 -> Product3/2
  Clock1/1 -> Product3/1, Product2/2
  Trigonometric Function2/1 -> Product1/2
  Constant3/1 -> Product2/1
  r/1 -> Product/2, Product1/1
  Product3/1 -> Sum/1
  Constant1/1 -> Sum/2

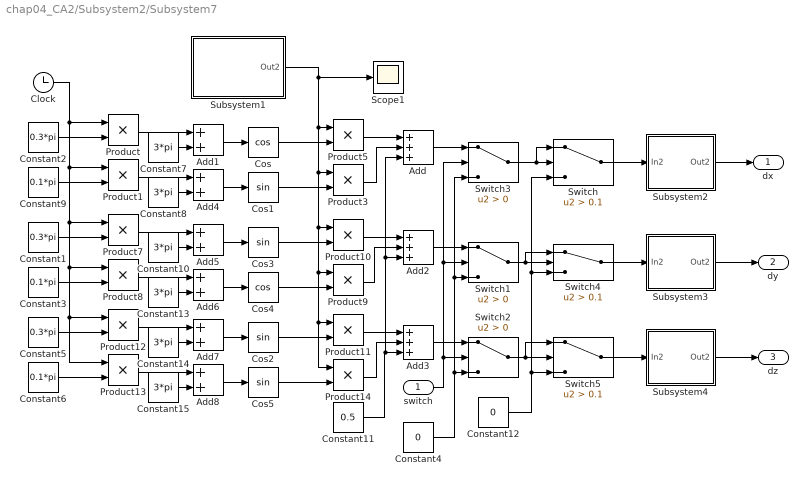
== system chap04_CA2/Subsystem2/Subsystem7 ==
  switch : Inport
  Add : Sum  Inputs=+++
  Add{1,4..8} (6 alike) : Sum
  Add2 : Sum  Inputs=+++
  Add3 : Sum  Inputs=+++
  Clock : Clock
  Constant1 : Constant  Value=0.3*pi
  Constant{7..8,10,13..15} (6 alike) : Constant  Value=3*pi
  Constant11 : Constant  Value=0.5
  Constant12 : Constant  Value=0
  Constant2 : Constant  Value=0.3*pi
  Constant3 : Constant  Value=0.1*pi
  Constant4 : Constant  Value=0
  Constant5 : Constant  Value=0.3*pi
  Constant6 : Constant  Value=0.1*pi
  Constant9 : Constant  Value=0.1*pi
  Cos : Trigonometry  Operator=cos
  Cos{1..3,5} (4 alike) : Trigonometry
  Cos4 : Trigonometry  Operator=cos
  Product{,1,3,5,7..14} (12 alike) : Product
  Scope1 : Scope
  Subsystem1 : Subsystem
  Subsystem2 : Subsystem
  Subsystem3 : Subsystem
  Subsystem4 : Subsystem
  Switch : Switch  Criteria=u2 > Threshold  Threshold=0.1
  Switch1 : Switch  Criteria=u2 > Threshold
  Switch2 : Switch  Criteria=u2 > Threshold
  Switch3 : Switch  Criteria=u2 > Threshold
  Switch4 : Switch  Criteria=u2 > Threshold  Threshold=0.1
  Switch5 : Switch  Criteria=u2 > Threshold  Threshold=0.1
  dx : Outport
  dy : Outport  Port=2
  dz : Outport  Port=3
  wires:
  Add/1 -> Switch3/1
  Add2/1 -> Switch1/1
  Switch2/1 -> Switch5/1, Switch5/2
  Product11/1 -> Add3/1
  Constant6/1 -> Product13/2
  Subsystem1/1(Out2) -> Scope1/1, Product11/1, Product14/1, Product9/1, Product10/1, Product3/1, Product5/1
  Product14/1 -> Add3/2
  Cos2/1 -> Product11/2
  Cos5/1 -> Product14/2
  Constant5/1 -> Product12/2
  Product12/1 -> Add7/1
  Product13/1 -> Add8/1
  Clock/1 -> Product/1, Product13/1, Product12/1, Product8/1, Product7/1, Product1/1
  Product10/1 -> Add2/1
  Product8/1 -> Add6/1
  Product7/1 -> Add5/1
  Constant1/1 -> Product7/2
  Cos4/1 -> Product9/2
  Cos3/1 -> Product10/2
  Product9/1 -> Add2/2
  Constant3/1 -> Product8/2
  Constant9/1 -> Product1/2
  Product3/1 -> Add/2
  Cos/1 -> Product5/2
  Add3/1 -> Switch2/1
  Cos1/1 -> Product3/2
  switch/1 -> Switch2/2, Switch1/2, Switch3/2
  Constant4/1 -> Switch3/3, Switch1/3, Switch2/3
  Product5/1 -> Add/1
  Constant2/1 -> Product/2
  Product/1 -> Add1/1
  Product1/1 -> Add4/1
  Switch1/1 -> Switch4/1, Switch4/2
  Switch3/1 -> Switch/1, Switch/2
  Switch/1 -> Subsystem2/1(In2)
  Constant12/1 -> Switch/3, Switch4/3, Switch5/3
  Constant11/1 -> Add/3, Add2/3, Add3/3
  Switch4/1 -> Subsystem3/1(In2)
  Switch5/1 -> Subsystem4/1(In2)
  Subsystem2/1(Out2) -> dx/1
  Subsystem3/1(Out2) -> dy/1
  Subsystem4/1(Out2) -> dz/1
  Add1/1 -> Cos/1
  Constant7/1 -> Add1/2
  Add4/1 -> Cos1/1
  Constant8/1 -> Add4/2
  Add5/1 -> Cos3/1
  Constant10/1 -> Add5/2
  Add6/1 -> Cos4/1
  Constant13/1 -> Add6/2
  Add7/1 -> Cos2/1
  Constant14/1 -> Add7/2
  Add8/1 -> Cos5/1
  Constant15/1 -> Add8/2

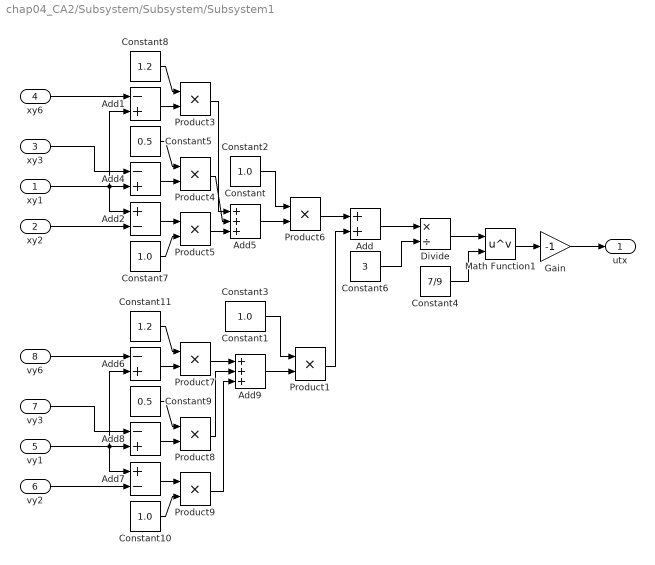
== system chap04_CA2/Subsystem/Subsystem/Subsystem1 ==
  xy1 : Inport
  xy2 : Inport  Port=2
  xy3 : Inport  Port=3
  xy6 : Inport  Port=4
  vy1 : Inport  Port=5
  vy2 : Inport  Port=6
  vy3 : Inport  Port=7
  vy6 : Inport  Port=8
  Add : Sum
  Add{1,4,6,8} (4 alike) : Sum  Inputs=-+
  Add2 : Sum  Inputs=+-
  Add5 : Sum  Inputs=+++
  Add7 : Sum  Inputs=+-
  Add9 : Sum  Inputs=+++
  Constant{,1..3,7,10} (6 alike) : Constant  Value=1.0
  Constant11 : Constant  Value=1.2
  Constant4 : Constant  Value=7/9
  Constant5 : Constant  Value=0.5
  Constant6 : Constant  Value=3
  Constant8 : Constant  Value=1.2
  Constant9 : Constant  Value=0.5
  Divide : Product  Inputs=*/
  Gain : Gain  Gain=-1
  Math Function1 : Math  Operator=pow  SignedPower=on  SaturateOnIntegerOverflow=on
  Product{1,3..9} (8 alike) : Product
  utx : Outport
  wires:
  Product8/1 -> Add9/2
  Product9/1 -> Add9/3
  Constant9/1 -> Product8/1
  Add8/1 -> Product8/2
  vy1/1 -> Add6/2, Add8/2, Add7/1
  Constant10/1 -> Product9/2
  Add7/1 -> Product9/1
  vy3/1 -> Add8/1
  vy2/1 -> Add7/2
  vy6/1 -> Add6/1
  Constant11/1 -> Product7/1
  Add6/1 -> Product7/2
  Product7/1 -> Add9/1
  Product3/1 -> Add5/1
  Add1/1 -> Product3/2
  Constant8/1 -> Product3/1
  xy6/1 -> Add1/1
  xy2/1 -> Add2/2
  xy3/1 -> Add4/1
  Add5/1 -> Product6/2
  Add2/1 -> Product5/1
  Product1/1 -> Add/2
  Product6/1 -> Add/1
  Constant7/1 -> Product5/2
  xy1/1 -> Add2/1, Add4/2, Add1/2
  Add4/1 -> Product4/2
  Constant5/1 -> Product4/1
  Product5/1 -> Add5/3
  Product4/1 -> Add5/2
  Add9/1 -> Product1/2
  Math Function1/1 -> Gain/1
  Constant6/1 -> Divide/2
  Divide/1 -> Math Function1/1
  Add/1 -> Divide/1
  Constant4/1 -> Math Function1/2
  Gain/1 -> utx/1
  Constant3/1 -> Product1/1
  Constant2/1 -> Product6/1

== system chap04_CA2/Subsystem/Subsystem/Subsystem10 ==
  utx : Inport
  uty : Inport  Port=2
  utz : Inport  Port=3
  Add : Sum
  Constant3 : Constant
  Constant4 : Constant  Value=0
  Data Store Memory : DataStoreMemory  DataStoreName=utkz1  ReadBeforeWriteMsg=warning  WriteAfterWriteMsg=warning  WriteAfterReadMsg=warning  ShowAdditionalParam=off
  Data Store Memory1 : DataStoreMemory  DataStoreName=utky1  ReadBeforeWriteMsg=warning  WriteAfterWriteMsg=warning  WriteAfterReadMsg=warning  ShowAdditionalParam=off
  Data Store Memory2 : DataStoreMemory  DataStoreName=utkx1  ReadBeforeWriteMsg=warning  WriteAfterWriteMsg=warning  WriteAfterReadMsg=warning  ShowAdditionalParam=off
  Data Store Memory3 : DataStoreMemory  DataStoreName=uc1  ReadBeforeWriteMsg=warning  WriteAfterWriteMsg=warning  WriteAfterReadMsg=warning  ShowAdditionalParam=off
  Data Store Read : DataStoreRead  DataStoreName=uc1  IndexOptions=Index vector (dialog)  Indices=1  OutputSizes=1
  Data Store Read4 : DataStoreRead  DataStoreName=utkx1  IndexOptions=Index vector (dialog)  Indices=1  OutputSizes=1
  Data Store Read5 : DataStoreRead  DataStoreName=utky1  IndexOptions=Index vector (dialog)  Indices=1  OutputSizes=1
  Data Store Read6 : DataStoreRead  DataStoreName=utkz1  IndexOptions=Index vector (dialog)  Indices=1  OutputSizes=1
  Data Store Write : DataStoreWrite  DataStoreName=uc1  IndexOptions=Index vector (dialog)  Indices=1  OutputSizes=1
  Data Store Write1 : DataStoreWrite  DataStoreName=utkx1  IndexOptions=Index vector (dialog)  Indices=1  OutputSizes=1
  Data Store Write2 : DataStoreWrite  DataStoreName=utky1  IndexOptions=Index vector (dialog)  Indices=1  OutputSizes=1
  Data Store Write6 : DataStoreWrite  DataStoreName=utkz1  IndexOptions=Index vector (dialog)  Indices=1  OutputSizes=1
  Demux : Demux  Outputs=3
  Display : Display
  MATLAB Function : MATLAB Function  TreatAsAtomicUnit=on
  Mux1 : Mux  Inputs=3
  Mux2 : Mux  Inputs=3
  Switch : Switch  Threshold=0.025
  Switch2 : Switch  Threshold=0.025
  ux : Outport
  uy : Outport  Port=2
  uz : Outport  Port=3
  wires:
  Switch/1 -> Demux/1
  Data Store Read4/1 -> Mux2/1
  Data Store Read6/1 -> Mux2/3
  Data Store Read5/1 -> Mux2/2
  Demux/3 -> Data Store Write6/1, uz/1
  Demux/1 -> Data Store Write1/1, ux/1
  Add/1 -> Data Store Write/1, Display/1
  Data Store Read/1 -> Add/2
  Switch2/1 -> Add/1  "e1"
  Constant3/1 -> Switch2/1
  Constant4/1 -> Switch2/3
  utx/1 -> Mux1/1
  uty/1 -> Mux1/2
  utz/1 -> Mux1/3
  Demux/2 -> Data Store Write2/1, uy/1
  [ut] -> Switch/1
  [utk] -> Switch/3
  MATLAB Function/1(nrom) -> Switch2/2, Switch/2
  Mux1/1 -> [ut], MATLAB Function/1(u)
  Mux2/1 -> [utk], MATLAB Function/2(utk)

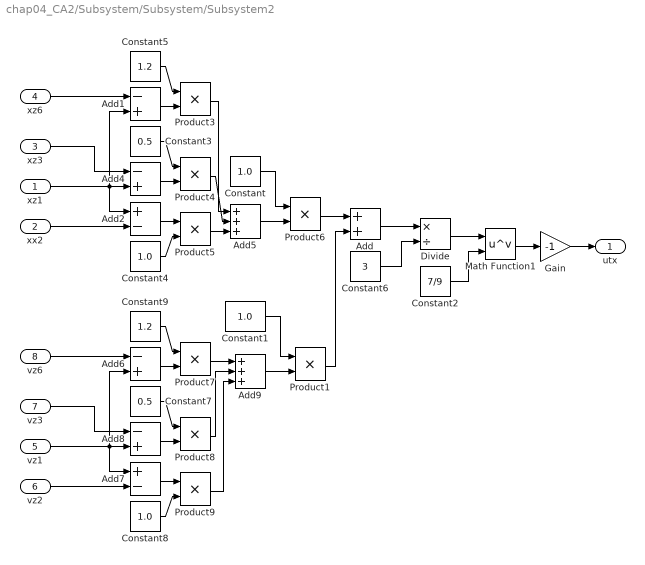
== system chap04_CA2/Subsystem/Subsystem/Subsystem2 ==
  xz1 : Inport
  xx2 : Inport  Port=2
  xz3 : Inport  Port=3
  xz6 : Inport  Port=4
  vz1 : Inport  Port=5
  vz2 : Inport  Port=6
  vz3 : Inport  Port=7
  vz6 : Inport  Port=8
  Add : Sum
  Add{1,4,6,8} (4 alike) : Sum  Inputs=-+
  Add2 : Sum  Inputs=+-
  Add5 : Sum  Inputs=+++
  Add7 : Sum  Inputs=+-
  Add9 : Sum  Inputs=+++
  Constant{,1,4,8} (4 alike) : Constant  Value=1.0
  Constant2 : Constant  Value=7/9
  Constant3 : Constant  Value=0.5
  Constant5 : Constant  Value=1.2
  Constant6 : Constant  Value=3
  Constant7 : Constant  Value=0.5
  Constant9 : Constant  Value=1.2
  Divide : Product  Inputs=*/
  Gain : Gain  Gain=-1
  Math Function1 : Math  Operator=pow  SignedPower=on  SaturateOnIntegerOverflow=on
  Product{1,3..9} (8 alike) : Product
  utx : Outport
  wires:
  Add9/1 -> Product1/2
  Product4/1 -> Add5/2
  Product5/1 -> Add5/3
  Constant3/1 -> Product4/1
  Add4/1 -> Product4/2
  xz1/1 -> Add1/2, Add4/2, Add2/1
  Constant4/1 -> Product5/2
  Product6/1 -> Add/1
  Constant/1 -> Product6/1
  Constant1/1 -> Product1/1
  Product1/1 -> Add/2
  Add2/1 -> Product5/1
  Add5/1 -> Product6/2
  xz3/1 -> Add4/1
  xx2/1 -> Add2/2
  xz6/1 -> Add1/1
  Constant5/1 -> Product3/1
  Add1/1 -> Product3/2
  Product3/1 -> Add5/1
  Product7/1 -> Add9/1
  Add6/1 -> Product7/2
  Constant9/1 -> Product7/1
  vz6/1 -> Add6/1
  vz2/1 -> Add7/2
  vz3/1 -> Add8/1
  Add7/1 -> Product9/1
  Constant8/1 -> Product9/2
  vz1/1 -> Add7/1, Add8/2, Add6/2
  Add8/1 -> Product8/2
  Constant7/1 -> Product8/1
  Product9/1 -> Add9/3
  Product8/1 -> Add9/2
  Math Function1/1 -> Gain/1
  Constant6/1 -> Divide/2
  Divide/1 -> Math Function1/1
  Add/1 -> Divide/1
  Constant2/1 -> Math Function1/2
  Gain/1 -> utx/1

== system chap04_CA2/Subsystem/Subsystem/Subsystem4 ==
  vx1 : Inport
  utx : Inport  Port=2
  gain : Inport  Port=3
  Add1 : Sum  Inputs=--+
  Constant : Constant  Value=0.08
  Constant2 : Constant  Value=15
  Product : Product
  Product1 : Product
  Product2 : Product
  Subsystem : Subsystem
  Subtract : Sum  Inputs=+-
  Tanh : Trigonometry  Operator=tanh
  ux : Outport
  wires:
  Add1/1 -> ux/1
  utx/1 -> [A], Subsystem/1(zt3)
  Subsystem/1(Out1) -> Subtract/2
  Product/1 -> Add1/2
  vx1/1 -> Subtract/1
  Product2/1 -> Tanh/1
  Tanh/1 -> Product/1
  gain/1 -> Product/2
  [A] -> Add1/3
  Constant2/1 -> Product2/2
  Product1/1 -> Add1/1
  Constant/1 -> Product1/1
  Subtract/1 -> Product1/2, Product2/1

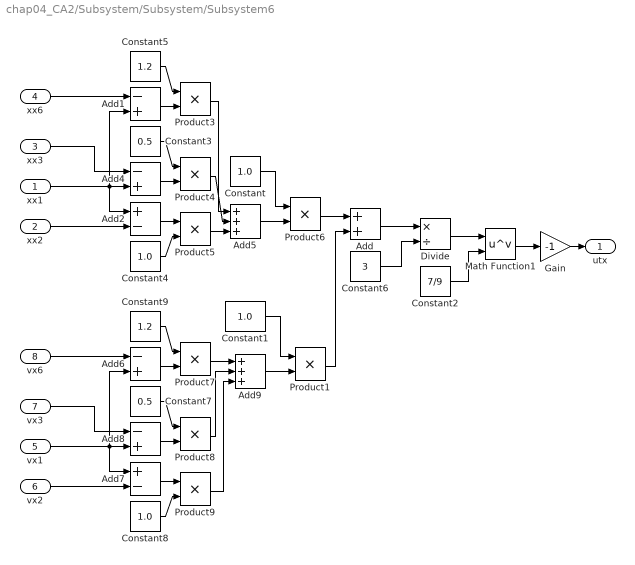
== system chap04_CA2/Subsystem/Subsystem/Subsystem6 ==
  xx1 : Inport
  xx2 : Inport  Port=2
  xx3 : Inport  Port=3
  xx6 : Inport  Port=4
  vx1 : Inport  Port=5
  vx2 : Inport  Port=6
  vx3 : Inport  Port=7
  vx6 : Inport  Port=8
  Add : Sum
  Add{1,4,6,8} (4 alike) : Sum  Inputs=-+
  Add2 : Sum  Inputs=+-
  Add5 : Sum  Inputs=+++
  Add7 : Sum  Inputs=+-
  Add9 : Sum  Inputs=+++
  Constant{,1,4,8} (4 alike) : Constant  Value=1.0
  Constant2 : Constant  Value=7/9
  Constant3 : Constant  Value=0.5
  Constant5 : Constant  Value=1.2
  Constant6 : Constant  Value=3
  Constant7 : Constant  Value=0.5
  Constant9 : Constant  Value=1.2
  Divide : Product  Inputs=*/
  Gain : Gain  Gain=-1
  Math Function1 : Math  Operator=pow  SignedPower=on  SaturateOnIntegerOverflow=on
  Product{1,3..9} (8 alike) : Product
  utx : Outport
  wires:
  Add9/1 -> Product1/2
  Product4/1 -> Add5/2
  Product5/1 -> Add5/3
  Constant3/1 -> Product4/1
  Add4/1 -> Product4/2
  xx1/1 -> Add1/2, Add4/2, Add2/1
  Constant4/1 -> Product5/2
  Product6/1 -> Add/1
  Constant/1 -> Product6/1
  Constant1/1 -> Product1/1
  Product1/1 -> Add/2
  Add2/1 -> Product5/1
  Add5/1 -> Product6/2
  xx3/1 -> Add4/1
  xx2/1 -> Add2/2
  xx6/1 -> Add1/1
  Constant5/1 -> Product3/1
  Add1/1 -> Product3/2
  Product3/1 -> Add5/1
  Product7/1 -> Add9/1
  Add6/1 -> Product7/2
  Constant9/1 -> Product7/1
  vx6/1 -> Add6/1
  vx2/1 -> Add7/2
  vx3/1 -> Add8/1
  Add7/1 -> Product9/1
  Constant8/1 -> Product9/2
  vx1/1 -> Add7/1, Add8/2, Add6/2
  Add8/1 -> Product8/2
  Constant7/1 -> Product8/1
  Product9/1 -> Add9/3
  Product8/1 -> Add9/2
  Gain/1 -> utx/1
  Constant2/1 -> Math Function1/2
  Add/1 -> Divide/1
  Math Function1/1 -> Gain/1
  Divide/1 -> Math Function1/1
  Constant6/1 -> Divide/2

== system chap04_CA2/Subsystem/Subsystem/Subsystem7 ==
  vy1 : Inport
  uty : Inport  Port=2
  gain : Inport  Port=3
  Add1 : Sum  Inputs=--+
  Constant : Constant  Value=0.08
  Constant2 : Constant  Value=15
  Product : Product
  Product1 : Product
  Product2 : Product
  Subsystem : Subsystem
  Subtract : Sum  Inputs=+-
  Tanh : Trigonometry  Operator=tanh
  ux : Outport
  wires:
  Subtract/1 -> Product2/1, Product1/2
  Constant/1 -> Product1/1
  Product1/1 -> Add1/1
  Constant2/1 -> Product2/2
  [A] -> Add1/3
  gain/1 -> Product/2
  Tanh/1 -> Product/1
  Product2/1 -> Tanh/1
  vy1/1 -> Subtract/1
  Product/1 -> Add1/2
  Subsystem/1(Out1) -> Subtract/2
  uty/1 -> Subsystem/1(zt3), [A]
  Add1/1 -> ux/1

== system chap04_CA2/Subsystem/Subsystem/Subsystem8 ==
  vz1 : Inport
  utz : Inport  Port=2
  gain : Inport  Port=3
  Add1 : Sum  Inputs=--+
  Constant : Constant  Value=0.08
  Constant2 : Constant  Value=15
  Product : Product
  Product1 : Product
  Product2 : Product
  Subsystem : Subsystem
  Subtract : Sum  Inputs=+-
  Tanh : Trigonometry  Operator=tanh
  ux : Outport
  wires:
  Add1/1 -> ux/1
  utz/1 -> [A], Subsystem/1(zt3)
  Subsystem/1(Out1) -> Subtract/2
  Product/1 -> Add1/2
  vz1/1 -> Subtract/1
  Product2/1 -> Tanh/1
  Tanh/1 -> Product/1
  gain/1 -> Product/2
  [A] -> Add1/3
  Constant2/1 -> Product2/2
  Product1/1 -> Add1/1
  Constant/1 -> Product1/1
  Subtract/1 -> Product1/2, Product2/1
